simulink model "Impcont_foot"  (R2016a)
settings: Solver=ode23tb  StartTime=0.0  StopTime=ti(end)  MaxStep=1e-3
InitFcn:
  | fp_sp_k = 12e3;
  | fp_sp_d = 1;
  | weights = 70/6;
  | joint_k = 0.1*180/pi;
  | joint_d = 1*180/pi;
  | fp_uj_dp_k = 500*180/pi;
  | fp_uj_dp_d = 1*180/pi;
  | fp_uj_ie_k = 500*180/pi;
  | fp_uj_ie_d = 1*180/pi;
  | 
  | x_k = 0*180/pi; x_d = 0.5*180/pi;
  | y_k = 0*180/pi; y_d = 0.5*180/pi;
  | z_k = 0*180/pi; z_d = 0.5*180/pi;
  | 
  | %{
  | stiff_dp=0.1*180/pi; stiff_ie=1*180/pi;
  | damp_dp=1*180/pi; damp_ie=1*180/pi;
  | % offset of prosthesis from centre of FP (XZY)
  |  sta=[-0.5345-6.54e-2 0.03779 0];
  | %}
  | 
  | % initpos = inv(jacob_gaitEmul(zeros(6,1)))*[ankle.trans(1,:).'; zeros(3,1)];
  | 
  | % sta = -[initpos(1) initpos(2) initpos(3)];
StopFcn:
  | %{
  | ankle = struct('ang_dp', angle_dp_out.signals.values,'ang_ie', angle_ie_out.signals.values,...
  |            'vel_dp',vel_dp.signals.values,'vel_ie',vel_ie.signals.values,...
  |            'acc_dp',acc_dp.signals.values,'acc_ie',acc_ie.signals.values,...
  |            'trans',ankle_trans_out.signals.values);
  | shin = struct('trans', trans_shin.signals.values, 'quat', quat_shin.signals.values);
  | foot = struct('trans', trans_foot.signals.values, 'quat', quat_foot.signals.values,...
  |     'acc',acc_foot.signals.values);
  | fplate = struct('trans', trans_fp.signals.values, 'quat', quat_fp.signals.values,...
  |     'torques', fp_torque_out.signals.values, 'forces', fp_force_out.signals.values);
  | 
  | [~, ~, ankle_ej.trans, ~] = est_joint(shin, foot);
  | 
  | fpForce = quatrotate(quatinv(fplate.quat), fplate.forces);
  | fpTorque = quatrotate(quatinv(fplate.quat), fplate.torques);
  | 
  | torque = cross(fplate.trans - ankle_ej.trans, fpForce) + fpTorque;
  | 
  | regMdl_dp = regress(torque(:,3),[ankle.ang_dp ankle.vel_dp foot.acc(:,3)]);
  | regMdl_ie = regress(torque(:,1),[ankle.ang_ie ankle.vel_ie foot.acc(:,1)]);
  | analysis_si = struct('kdp',regMdl_dp(1),'bdp',regMdl_dp(2),...
  |     'kie',regMdl_ie(1),'bie',regMdl_ie(2),'Jdp',regMdl_dp(3),...
  |     'Jie',regMdl_ie(3));
  | 
  | % %{
  | regMdl_dp = regress(torque(:,3),[ankle.ang_dp ankle.vel_dp ankle.acc_dp]);
  | regMdl_ie = regress(torque(:,1),[ankle.ang_ie ankle.vel_ie ankle.acc_ie]);
  | analysis_si2 = struct('kdp',regMdl_dp(1),'bdp',regMdl_dp(2),...
  |     'kie',regMdl_ie(1),'bie',regMdl_ie(2),'Jdp',regMdl_dp(3),...
  |     'Jie',regMdl_ie(3));
  | % %}
  | 
  | % %{
  | regMdl_dp = regress(tt_dp.signals.values(:,3),[ankle.ang_dp ankle.vel_dp ankle.acc_dp]);
  | regMdl_ie = regress(tt_ie.signals.values(:,3),[ankle.ang_ie ankle.vel_ie ankle.acc_ie]);
  | analysis_si3 = struct('kdp',regMdl_dp(1),'bdp',regMdl_dp(2),...
  |     'kie',regMdl_ie(1),'bie',regMdl_ie(2),'Jdp',regMdl_dp(3),...
  |     'Jie',regMdl_ie(3));
  | % %}
  | 
  | % %{
  | regMdl_dp = regress(tt_dp.signals.values(:,3),[ankle.ang_dp ankle.vel_dp foot.acc(:,3)]);
  | regMdl_ie = regress(tt_ie.signals.values(:,3),[ankle.ang_ie ankle.vel_ie foot.acc(:,1)]);
  | analysis_si4 = struct('kdp',regMdl_dp(1),'bdp',regMdl_dp(2),...
  |     'kie',regMdl_ie(1),'bie',regMdl_ie(2),'Jdp',regMdl_dp(3),...
  |     'Jie',regMdl_ie(3));
  | % %}
  | 
  | regMdl_dp = regress(torque(:,3),[ankle.ang_dp ankle.vel_dp]);
  | regMdl_ie = regress(torque(:,1),[ankle.ang_ie ankle.vel_ie]);
  | analysis_si5 = struct('kdp',regMdl_dp(1),'bdp',regMdl_dp(2),...
  |     'kie',regMdl_ie(1),'bie',regMdl_ie(2));
  | 
  | %}
values from neighbouring files (symbols this model uses):
  N = length(shin_angles_in.signals.values)    [GaitEmu_code.m]    (also in dy1.m; dy2.m; est_joint.m = size( [body1.trans body2.trans], 1 ); impcont.m)
  s = [-atan((t2.*3.379e-4+t3+t4.*t5.*4.401e-2)./(t4.*cos(q2)));-asin(t2.*1.4870979e-5+t3.*4.401e-2-t4.*t5)]    [FK_af.m]    (also in FK_footimp.m = [atan((ree2_1.*t2.*4.401e-2+ree2_2.*t4+ree2_3.*t3+t5.*t7.*4.; FK_gaitEmul.m = [q1+t2.*t4.*4.234e-1+t3.*t5.*1.5e-3-t2.*t6.*t7.*1.5e-3-5.347; ik.m = [x; y; z]; ik_af.m = FK_af(q))
  Y = -( reshape( body1.trans', [], 1 ) - reshape( body2.trans', [], 1 ) )    [creat_joint.m]    (also in est_joint.m = -( reshape( body1.trans', [3*N 1] ) - reshape( body2.trans',)
undefined symbols (not defined in the file or in its folder): X, Z
libraries: sm_lib x274, nesl_utility x100, simulink x3, dspstat3 x2, aerolibtransform2 x1
(part 1 of 7)
settings Model: Creator=lcasteli  LastModifiedBy=lcasteli
settings SolverCC: ZeroCrossControl=DisableAll  AlgebraicLoopSolver=LineSearch
settings DataIOCC: OutputTimes=[0:0.01:t(end)]
settings ModelReferenceCC: ModelReferenceMinAlgLoopOccurrences=on

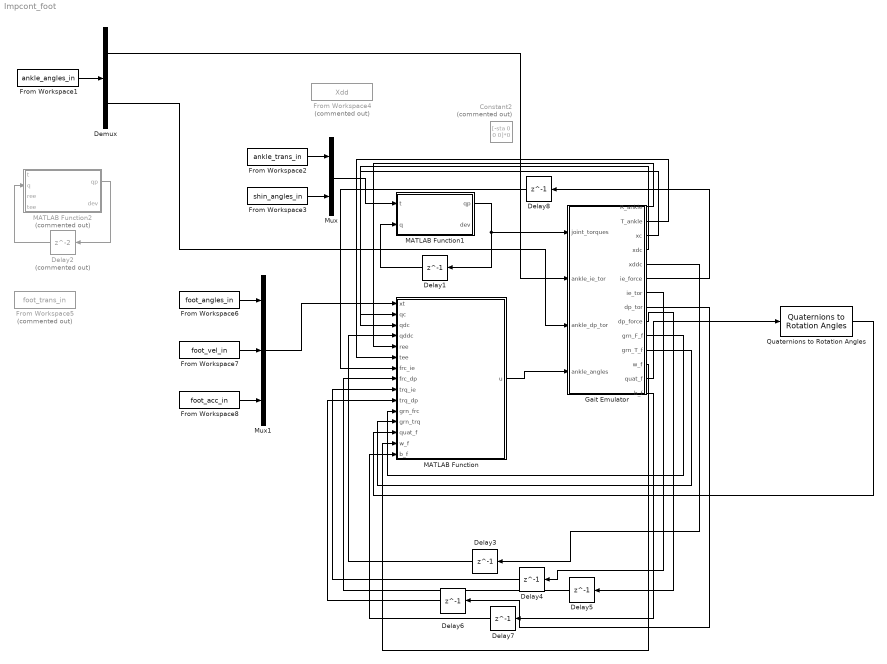
== system Impcont_foot ==
  Constant2 : Constant  Commented=on  Value=[-sta 0 0 0]*0
  Delay{1,3..8} (7 alike) : Delay  DelayLength=1  SampleTime=0.01
  Delay2 : Delay  Commented=on  SampleTime=0.01
  Demux : Demux  Outputs=2
  From Workspace1 : FromWorkspace  VariableName=ankle_angles_in  SampleTime=0
  From Workspace2 : FromWorkspace  VariableName=ankle_trans_in  SampleTime=0
  From Workspace3 : FromWorkspace  VariableName=shin_angles_in  SampleTime=0
  From Workspace4 : FromWorkspace  Commented=on  VariableName=Xdd  SampleTime=0
  From Workspace5 : FromWorkspace  Commented=on  VariableName=foot_trans_in  SampleTime=0
  From Workspace6 : FromWorkspace  VariableName=foot_angles_in  SampleTime=0
  From Workspace7 : FromWorkspace  VariableName=foot_vel_in  SampleTime=0
  From Workspace8 : FromWorkspace  VariableName=foot_acc_in  SampleTime=0
  Gait Emulator : Subsystem
  MATLAB Function : MATLAB Function  TreatAsAtomicUnit=on
  MATLAB Function1 : MATLAB Function  TreatAsAtomicUnit=on
  MATLAB Function2 : MATLAB Function  Commented=on  TreatAsAtomicUnit=on
  Mux : Mux  Inputs=2
  Mux1 : Mux  Inputs=3
  Quaternions to Rotation Angles : aerolibtransform2/Quaternions to Rotation Angles  rotationOrder=XYZ
  wires:
  Delay1/1 -> MATLAB Function1/2(q)
  MATLAB Function1/1(qp) -> Delay1/1, Gait Emulator/1(joint_torques)
  From Workspace1/1 -> Demux/1
  From Workspace2/1 -> Mux/1
  From Workspace3/1 -> Mux/2
  Mux/1 -> MATLAB Function1/1(t)
  Gait Emulator/2(T_ankle) -> MATLAB Function/6(tee)
  Gait Emulator/1(R_ankle) -> MATLAB Function/5(ree)
  Gait Emulator/3(xc) -> MATLAB Function/2(qc)
  Gait Emulator/4(xdc) -> MATLAB Function/3(qdc)
  Gait Emulator/5(xddc) -> Delay3/1
  Gait Emulator/6(ie_force) -> Delay8/1
  Gait Emulator/7(ie_tor) -> Delay4/1
  Gait Emulator/9(dp_force) -> Delay5/1
  Gait Emulator/8(dp_tor) -> Delay6/1
  MATLAB Function2/1(qp) -> Delay2/1
  Delay2/1 -> MATLAB Function2/2(q)
  From Workspace8/1 -> Mux1/3
  From Workspace7/1 -> Mux1/2
  From Workspace6/1 -> Mux1/1
  Mux1/1 -> MATLAB Function/1(xt)
  MATLAB Function/1(u) -> Gait Emulator/4(ankle_angles)
  Gait Emulator/10(grn_F_f) -> MATLAB Function/11(grn_frc)
  Gait Emulator/11(grn_T_f) -> MATLAB Function/12(grn_trq)
  Gait Emulator/14(b_f) -> Delay7/1
  Gait Emulator/13(quat_f) -> Quaternions to Rotation Angles/1
  Quaternions to Rotation Angles/1 -> MATLAB Function/13(quat_f)
  Delay3/1 -> MATLAB Function/4(qddc)
  Delay4/1 -> MATLAB Function/9(trq_ie)
  Delay5/1 -> MATLAB Function/8(frc_dp)
  Delay6/1 -> MATLAB Function/10(trq_dp)
  Delay7/1 -> MATLAB Function/15(b_f)
  Gait Emulator/12(w_f) -> MATLAB Function/14(w_f)
  Delay8/1 -> MATLAB Function/7(frc_ie)
  Demux/1 -> Gait Emulator/2(ankle_ie_tor)
  Demux/2 -> Gait Emulator/3(ankle_dp_tor)

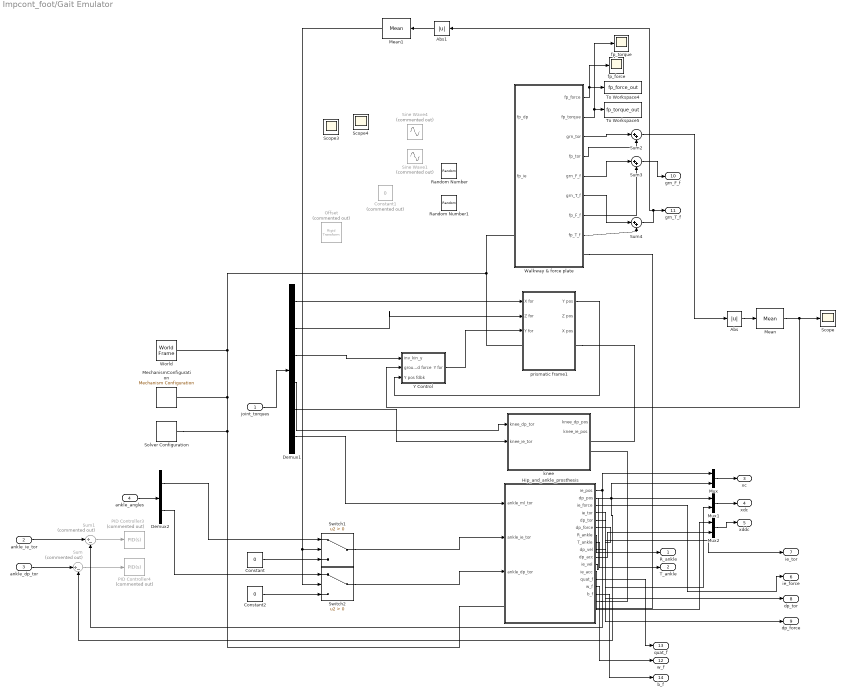
== system Impcont_foot/Gait Emulator ==
  joint_torques : Inport
  ankle_ie_tor : Inport  Port=2
  ankle_dp_tor : Inport  Port=3
  ankle_angles : Inport  Port=4
  Abs : Abs
  Abs1 : Abs
  Constant : Constant  Value=0
  Constant1 : Constant  Commented=on  Value=0
  Constant2 : Constant  Value=0
  Demux1 : Demux  Outputs=6
  Demux2 : Demux  Outputs=2
  Hip_and_ankle_prosthesis : Subsystem
  Mean : dspstat3/Mean  run=off  reset_popup=None  InputProcessing=Columns as channels (frame based)  directionMode=Each column  dimension=1  roiEnable=off  roiType=Rectangles  roiPortion=Entire ROI  roiOutput=Individual statistics for each ROI  roiFlag=off  outputDataTypeStr=Inherit: Same as accumulator  outputLastDataTypeStr=Inherit: Same as accumulator  outputMin=[]  outputMax=[]  roundingMode=Floor  overflowMode=off
  Mean1 : dspstat3/Mean  run=off  reset_popup=None  InputProcessing=Columns as channels (frame based)  directionMode=Each column  dimension=1  roiEnable=off  roiType=Rectangles  roiPortion=Entire ROI  roiOutput=Individual statistics for each ROI  roiFlag=off  outputDataTypeStr=Inherit: Same as accumulator  outputLastDataTypeStr=Inherit: Same as accumulator  outputMin=[]  outputMax=[]  roundingMode=Floor  overflowMode=off
  MechanismConfiguration : sm_lib/Utilities/Mechanism Configuration  UniformGravity=Constant  GravityVector=[0 -9.81 0]  GravityUnits=m/s^2  LinearizationDelta=0.001
  Mux : Mux  Inputs=2
  Mux1 : Mux  Inputs=2
  Mux2 : Mux  Inputs=2
  Offset : sm_lib/Frames and Transforms/Rigid Transform  Commented=on  TranslationMethod=Cartesian  TranslationLengthUnit=m  TranslationStandardAxis=+Z  TranslationStandardOffset=0  TranslationCartesianOffset=[0.5345 0 -0.03779]  TranslationROffset=0  TranslationROffsetUnits=m  TranslationZOffset=0  TranslationZOffsetUnits=m  TranslationThetaOffset=0  TranslationThetaOffsetUnits=deg  RotationMethod=None  RotationAngleUnits=deg  RotationStandardAxis=+Z  RotationAngle=0.0  RotationArbitraryAxis=[0 0 1]  FollAlignAxisA=+X  BaseAlignAxisA=+Y  FollAlignAxisB=+Y  BaseAlignAxisB=+Z  RotationSequenceAxes=FollowerAxes  RotationSequence=XYX  RotationSequenceAngles=[0 0 0]  RotationSequenceAnglesUnits=deg  RotationMatrix=[1 0 0; 0 1 0; 0 0 1]
  PID Controller3 : simulink/Continuous/PID Controller  Commented=on  Controller=PID  TimeDomain=Continuous-time  SampleTime=-1  IntegratorMethod=Forward Euler  FilterMethod=Forward Euler  Form=Parallel  UseFilter=on  ControllerParametersSource=internal  P=975.875057621142  I=4739.46701283172  D=-0.483288607910801  N=2019.23869432746  InitialConditionSource=internal  InitialConditionForIntegrator=0  InitialConditionForFilter=0  ExternalReset=none  LimitOutput=off  UpperSaturationLimit=300  LowerSaturationLimit=-300  LinearizeAsGain=on  AntiWindupMode=clamping  Kb=1  TrackingMode=off  Kt=1  PParamMin=[]  PParamMax=[]  IParamMin=[]  IParamMax=[]  DParamMin=[]  DParamMax=[]  NParamMin=[]  NParamMax=[]  KbParamMin=[]  KbParamMax=[]  KtParamMin=[]  KtParamMax=[]  POutMin=[]  POutMax=[]  IOutMin=[]  IOutMax=[]  DOutMin=[]  DOutMax=[]  NOutMin=[]  NOutMax=[]  KbOutMin=[]  KbOutMax=[]  KtOutMin=[]  KtOutMax=[]  IntegratorOutMin=[]  IntegratorOutMax=[]  FilterOutMin=[]  FilterOutMax=[]  SumOutMin=[]  SumOutMax=[]  SumI1OutMin=[]  SumI1OutMax=[]  SumI2OutMin=[]  SumI2OutMax=[]  SumI3OutMin=[]  SumI3OutMax=[]  SumDOutMin=[]  SumDOutMax=[]  SaturationOutMin=[]  SaturationOutMax=[]  IntegratorContinuousStateAttributes=''  IntegratorStateMustResolveToSignalObject=off  IntegratorRTWStateStorageClass=Auto  FilterContinuousStateAttributes=''  FilterStateMustResolveToSignalObject=off  FilterRTWStateStorageClass=Auto  DifferentiatorICPrevScaledInput=0  DifferentiatorOutMin=[]  DifferentiatorOutMax=[]
  PID Controller4 : simulink/Continuous/PID Controller  Commented=on  Controller=PID  TimeDomain=Continuous-time  SampleTime=-1  IntegratorMethod=Forward Euler  FilterMethod=Forward Euler  Form=Parallel  UseFilter=on  ControllerParametersSource=internal  P=1292.14032707455  I=5309.73525196698  D=-11.9075203483279  N=25.559430935789  InitialConditionSource=internal  InitialConditionForIntegrator=0  InitialConditionForFilter=0  ExternalReset=none  LimitOutput=off  UpperSaturationLimit=300  LowerSaturationLimit=-300  LinearizeAsGain=on  AntiWindupMode=clamping  Kb=1  TrackingMode=off  Kt=1  PParamMin=[]  PParamMax=[]  IParamMin=[]  IParamMax=[]  DParamMin=[]  DParamMax=[]  NParamMin=[]  NParamMax=[]  KbParamMin=[]  KbParamMax=[]  KtParamMin=[]  KtParamMax=[]  POutMin=[]  POutMax=[]  IOutMin=[]  IOutMax=[]  DOutMin=[]  DOutMax=[]  NOutMin=[]  NOutMax=[]  KbOutMin=[]  KbOutMax=[]  KtOutMin=[]  KtOutMax=[]  IntegratorOutMin=[]  IntegratorOutMax=[]  FilterOutMin=[]  FilterOutMax=[]  SumOutMin=[]  SumOutMax=[]  SumI1OutMin=[]  SumI1OutMax=[]  SumI2OutMin=[]  SumI2OutMax=[]  SumI3OutMin=[]  SumI3OutMax=[]  SumDOutMin=[]  SumDOutMax=[]  SaturationOutMin=[]  SaturationOutMax=[]  IntegratorContinuousStateAttributes=''  IntegratorStateMustResolveToSignalObject=off  IntegratorRTWStateStorageClass=Auto  FilterContinuousStateAttributes=''  FilterStateMustResolveToSignalObject=off  FilterRTWStateStorageClass=Auto  DifferentiatorICPrevScaledInput=0  DifferentiatorOutMin=[]  DifferentiatorOutMax=[]
  Random Number : RandomNumber  Variance=4e5  SampleTime=0.1
  Random Number1 : RandomNumber  Variance=1e4  SampleTime=0.1
  Scope : Scope
  Scope3 : Scope
  Scope4 : Scope
  Sine Wave1 : Sin  Commented=on  Amplitude=100  Frequency=10  Phase=pi/6  SampleTime=0.001
  Sine Wave4 : Sin  Commented=on  Amplitude=100*2  Frequency=10  SampleTime=0.001
  Solver Configuration : nesl_utility/Solver Configuration  PhysicalDomain=network_engine_domain  SubClassName=solver  LeftPortType=input  RightPortType=generic  Accelerate=off  Tones=[]  Harmonics=[]  SimulateNoise=off  Profile=off  UseLocalSampling=off  EnableSwitchedLinearOptims=on  FrequencyDomain=off  UseCCode=off  RelTol=0.001  AbsTol=1e-06  MinStep=1e-09  ToWorkspace=off  RevertToSquareIcSolve=off  NumHomotopyIterations=100  PhasorMode=off  PhasorModeNumHarmonics=1  OverrideAbsTol=off  DoDC=off  ResidualTolerance=1e-09  UseLocalSolver=off  LocalSolverChoice=NE_BACKWARD_EULER_ADVANCER  LocalSolverSampleTime=0.001  DoFixedCost=off  MaxNonlinIter=3  MaxModeIter=2  LinearAlgebra=Sparse  DelaysMemoryBudget=1024  AutomaticFiltering=on  FilteringTimeConstant=0.001
  Sum : Sum  Commented=on  Inputs=|+-
  Sum1 : Sum  Commented=on  Inputs=|+-
  Sum2 : Sum  Inputs=|++
  Sum3 : Sum  Inputs=|++
  Sum4 : Sum  Inputs=|++
  Switch1 : Switch  Criteria=u2 > Threshold
  Switch2 : Switch  Criteria=u2 > Threshold
  To Workspace4 : ToWorkspace  VariableName=fp_force_out  SaveFormat=Structure With Time  SampleTime=-1
  To Workspace5 : ToWorkspace  VariableName=fp_torque_out  SaveFormat=Structure With Time  SampleTime=-1
  Walkway & force plate : Subsystem
  World : sm_lib/Frames and Transforms/World Frame
  Y Control : Subsystem
  fp_force : Scope
  fp_torque : Scope
  "knee " : Subsystem
  prismatic frame1 : Subsystem
  R_ankle : Outport
  T_ankle : Outport  Port=2
  xc : Outport  Port=3
  xdc : Outport  Port=4
  xddc : Outport  Port=5
  ie_force : Outport  Port=6
  ie_tor : Outport  Port=7
  dp_tor : Outport  Port=8
  dp_force : Outport  Port=9
  grn_F_f : Outport  Port=10
  grn_T_f : Outport  Port=11
  w_f : Outport  Port=12
  quat_f : Outport  Port=13
  b_f : Outport  Port=14
  wires:
  joint_torques/1 -> Demux1/1
  Walkway & force plate/2(fp_torque) -> fp_torque/1, To Workspace5/1
  Walkway & force plate/1(fp_force) -> To Workspace4/1, fp_force/1
  Demux1/4 -> "knee "/1(knee_dp_tor)
  Demux1/5 -> "knee "/2(knee_ie_tor)
  Demux1/6 -> Hip_and_ankle_prosthesis/1(ankle_ml_tor)
  Walkway & force plate/3(grn_tor) -> Sum2/1
  Walkway & force plate/4(fp_tor) -> Sum2/2
  Sum2/1 -> Abs/1
  Abs/1 -> Mean/1
  Mean/1 -> Y Control/2(ground force), Scope/1
  Hip_and_ankle_prosthesis/2(dp_pos) -> Sum/2, Mux/2
  Sum1/1 -> PID Controller3/1
  Sum/1 -> PID Controller4/1
  Demux1/1 -> prismatic frame1/1(X for)
  prismatic frame1/1(Y pos) -> Y Control/3(Y pos fdbk)
  Demux1/2 -> prismatic frame1/2(Z for)
  Demux1/3 -> Y Control/1(inv_kin_y)
  Y Control/1(Y for) -> prismatic frame1/3(Y for)
  ankle_ie_tor/1 -> Sum1/1
  ankle_dp_tor/1 -> Sum/1
  Hip_and_ankle_prosthesis/8(T_ankle) -> T_ankle/1
  Hip_and_ankle_prosthesis/7(R_ankle) -> R_ankle/1
  ankle_angles/1 -> Demux2/1
  Hip_and_ankle_prosthesis/1(ie_pos) -> Sum1/2, Mux/1
  Hip_and_ankle_prosthesis/11(ie_vel) -> Mux1/1
  Hip_and_ankle_prosthesis/9(dp_vel) -> Mux1/2
  Hip_and_ankle_prosthesis/12(ie_acc) -> Mux2/1
  Hip_and_ankle_prosthesis/10(dp_acc) -> Mux2/2
  Mux2/1 -> xddc/1
  Mux1/1 -> xdc/1
  Mux/1 -> xc/1
  Hip_and_ankle_prosthesis/3(ie_force) -> ie_force/1
  Hip_and_ankle_prosthesis/4(ie_tor) -> ie_tor/1
  Hip_and_ankle_prosthesis/6(dp_force) -> dp_force/1
  Hip_and_ankle_prosthesis/5(dp_tor) -> dp_tor/1
  Sum3/1 -> grn_F_f/1
  Hip_and_ankle_prosthesis/13(quat_f) -> quat_f/1
  Hip_and_ankle_prosthesis/14(w_f) -> w_f/1
  Hip_and_ankle_prosthesis/15(b_f) -> b_f/1
  Walkway & force plate/7(fp_F_f) -> Sum3/2
  Walkway & force plate/5(grn_F_f) -> Sum3/1
  Walkway & force plate/8(fp_T_f) -> Sum4/2
  Walkway & force plate/6(grn_T_f) -> Sum4/1
  Sum4/1 -> grn_T_f/1, Abs1/1
  Demux2/1 -> Switch1/1
  Demux2/2 -> Switch2/1
  Switch1/1 -> Hip_and_ankle_prosthesis/2(ankle_ie_tor)
  Switch2/1 -> Hip_and_ankle_prosthesis/3(ankle_dp_tor)
  Abs1/1 -> Mean1/1
  Mean1/1 -> Switch2/2, Switch1/2
  Constant2/1 -> Switch2/3
  Constant/1 -> Switch1/3
  connections:
  Hip_and_ankle_prosthesis/RConn1 -- "knee "/RConn2
  Walkway & force plate/RConn1 -- Hip_and_ankle_prosthesis/RConn2
  prismatic frame1/LConn1 -- Walkway & force plate/LConn1 -- Hip_and_ankle_prosthesis/LConn1 -- Solver Configuration/RConn1 -- MechanismConfiguration/RConn1 -- World/RConn1
  prismatic frame1/RConn1 -- "knee "/RConn1

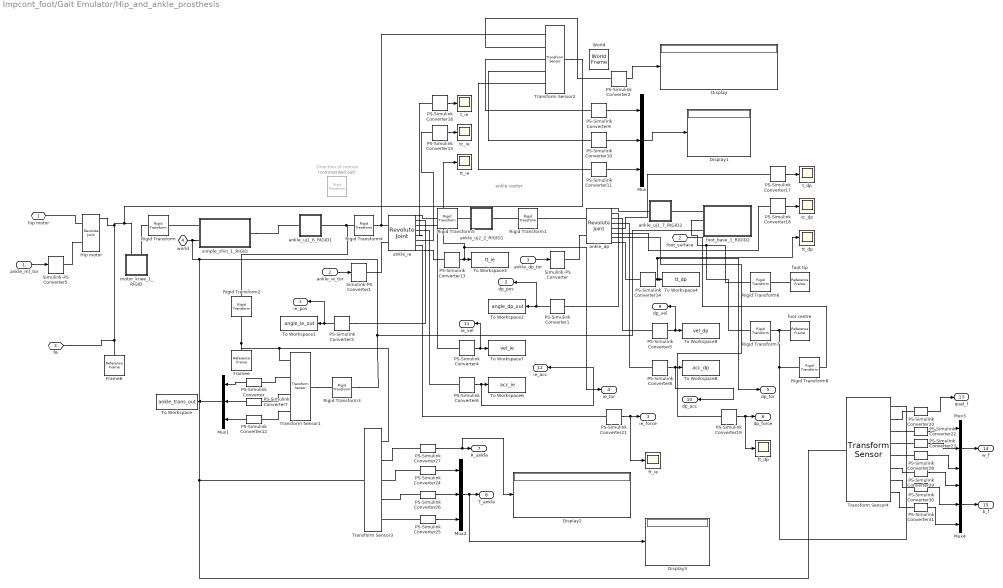
== system Impcont_foot/Gait Emulator/Hip_and_ankle_prosthesis ==
  note: ankle center
  ankle_ml_tor : Inport
  ankle_ie_tor : Inport  Port=2
  ankle_dp_tor : Inport  Port=3
  Display{,1..3} (4 alike) : Display
  Driection of motion : sm_lib/Frames and Transforms/Rigid Transform  Commented=on  TranslationMethod=None  TranslationLengthUnit=m  TranslationStandardAxis=+Z  TranslationStandardOffset=0  TranslationCartesianOffset=[0 0 0]  TranslationROffset=0  TranslationROffsetUnits=m  TranslationZOffset=0  TranslationZOffsetUnits=m  TranslationThetaOffset=0  TranslationThetaOffsetUnits=deg  RotationMethod=StandardAxis  RotationAngleUnits=deg  RotationStandardAxis=+Z  RotationAngle=0  RotationArbitraryAxis=[0 0 1]  FollAlignAxisA=+X  BaseAlignAxisA=+Y  FollAlignAxisB=+Y  BaseAlignAxisB=+Z  RotationSequenceAxes=FollowerAxes  RotationSequence=XYX  RotationSequenceAngles=[0 0 0]  RotationSequenceAnglesUnits=deg  RotationMatrix=[1 0 0; 0 1 0; 0 0 1]
  Frame6 : sm_lib/Frames and Transforms/Reference Frame
  Framee : sm_lib/Frames and Transforms/Reference Frame
  Hip motor : sm_lib/Joints/Revolute Joint  SenseConstraintForce=off  SenseConstraintForceX=off  SenseConstraintForceY=off  SenseConstraintForceZ=off  SenseConstraintTorque=off  SenseConstraintTorqueX=off  SenseConstraintTorqueY=off  SenseConstraintTorqueZ=off  SenseTotalForce=on  SenseTotalForceX=off  SenseTotalForceY=off  SenseTotalForceZ=off  SenseTotalTorque=on  SenseTotalTorqueX=off  SenseTotalTorqueY=off  SenseTotalTorqueZ=off  CompositeWrenchDir=FollowerOnBase  CompositeWrenchFrame=BaseFrame  EquilibriumPosition=0  EquilibriumPositionUnits=rad  SpringStiffness=joint_k  SpringStiffnessUnits=m*N/rad  DampingCoefficient=joint_d  DampingCoefficientUnits=m*s*N/rad  TorqueActuationMode=ComputedTorque  MotionActuationMode=InputMotion  SensePosition=on  SenseVelocity=off  SenseAcceleration=off  SenseTorqueForce=off  PositionTargetSpecify=off  PositionTargetPriority=Low  PositionTargetValue=0  PositionTargetValueUnits=deg  VelocityTargetSpecify=off  VelocityTargetPriority=High  VelocityTargetValue=0  VelocityTargetValueUnits=deg/s
  Mux{,1..4} (5 alike) : Mux  Inputs=3
  PS-Simulink Converter{,1..31} (32 alike) : nesl_utility/PS-Simulink Converter  PhysicalDomain=network_engine_domain  SubClassName=ps_output  LeftPortType=input  RightPortType=output  PseudoPeriodic=off  Frequencies=[]  Unit=1  AffineConversion=off
  Rigid Transform : sm_lib/Frames and Transforms/Rigid Transform  TranslationMethod=StandardAxis  TranslationLengthUnit=m  TranslationStandardAxis=+Z  TranslationStandardOffset=0.15  TranslationCartesianOffset=[0 0 0]  TranslationROffset=0  TranslationROffsetUnits=m  TranslationZOffset=0  TranslationZOffsetUnits=m  TranslationThetaOffset=0  TranslationThetaOffsetUnits=deg  RotationMethod=StandardAxis  RotationAngleUnits=deg  RotationStandardAxis=+X  RotationAngle=180  RotationArbitraryAxis=[1 0 1]  FollAlignAxisA=+X  BaseAlignAxisA=+Y  FollAlignAxisB=+Y  BaseAlignAxisB=+Z  RotationSequenceAxes=FollowerAxes  RotationSequence=XYX  RotationSequenceAngles=[0 0 0]  RotationSequenceAnglesUnits=deg  RotationMatrix=[1 0 0; 0 1 0; 0 0 1]
  Rigid Transform1 : sm_lib/Frames and Transforms/Rigid Transform  TranslationMethod=None  TranslationLengthUnit=m  TranslationStandardAxis=+Z  TranslationStandardOffset=0.15  TranslationCartesianOffset=[0 0 0]  TranslationROffset=0  TranslationROffsetUnits=m  TranslationZOffset=0  TranslationZOffsetUnits=m  TranslationThetaOffset=0  TranslationThetaOffsetUnits=deg  RotationMethod=StandardAxis  RotationAngleUnits=deg  RotationStandardAxis=+Z  RotationAngle=-90  RotationArbitraryAxis=[1 0 1]  FollAlignAxisA=+X  BaseAlignAxisA=+Y  FollAlignAxisB=+Y  BaseAlignAxisB=+Z  RotationSequenceAxes=FollowerAxes  RotationSequence=XYX  RotationSequenceAngles=[0 0 0]  RotationSequenceAnglesUnits=deg  RotationMatrix=[1 0 0; 0 1 0; 0 0 1]
  Rigid Transform2 : sm_lib/Frames and Transforms/Rigid Transform  TranslationMethod=StandardAxis  TranslationLengthUnit=m  TranslationStandardAxis=+Z  TranslationStandardOffset=-8.5e-3  TranslationCartesianOffset=[0 0 0]  TranslationROffset=0  TranslationROffsetUnits=m  TranslationZOffset=0  TranslationZOffsetUnits=m  TranslationThetaOffset=0  TranslationThetaOffsetUnits=deg  RotationMethod=AlignedAxes  RotationAngleUnits=deg  RotationStandardAxis=+Z  RotationAngle=-90  RotationArbitraryAxis=[1 0 1]  FollAlignAxisA=+X  BaseAlignAxisA=-Z  FollAlignAxisB=+Y  BaseAlignAxisB=-Y  RotationSequenceAxes=FollowerAxes  RotationSequence=XYX  RotationSequenceAngles=[0 0 0]  RotationSequenceAnglesUnits=deg  RotationMatrix=[1 0 0; 0 1 0; 0 0 1]
  Rigid Transform3 : sm_lib/Frames and Transforms/Rigid Transform  TranslationMethod=StandardAxis  TranslationLengthUnit=m  TranslationStandardAxis=+Y  TranslationStandardOffset=0.1517  TranslationCartesianOffset=[0 0 0]  TranslationROffset=0  TranslationROffsetUnits=m  TranslationZOffset=0  TranslationZOffsetUnits=m  TranslationThetaOffset=0  TranslationThetaOffsetUnits=deg  RotationMethod=None  RotationAngleUnits=deg  RotationStandardAxis=+Z  RotationAngle=0.0  RotationArbitraryAxis=[0 0 1]  FollAlignAxisA=+X  BaseAlignAxisA=+Y  FollAlignAxisB=+Y  BaseAlignAxisB=+Z  RotationSequenceAxes=FollowerAxes  RotationSequence=XYX  RotationSequenceAngles=[0 0 0]  RotationSequenceAnglesUnits=deg  RotationMatrix=[1 0 0; 0 1 0; 0 0 1]
  Rigid Transform4 : sm_lib/Frames and Transforms/Rigid Transform  TranslationMethod=StandardAxis  TranslationLengthUnit=m  TranslationStandardAxis=+Z  TranslationStandardOffset=-8.5e-3  TranslationCartesianOffset=[0 0 0]  TranslationROffset=0  TranslationROffsetUnits=m  TranslationZOffset=0  TranslationZOffsetUnits=m  TranslationThetaOffset=0  TranslationThetaOffsetUnits=deg  RotationMethod=None  RotationAngleUnits=deg  RotationStandardAxis=+Z  RotationAngle=0.0  RotationArbitraryAxis=[0 0 1]  FollAlignAxisA=+X  BaseAlignAxisA=+Y  FollAlignAxisB=+Y  BaseAlignAxisB=+Z  RotationSequenceAxes=FollowerAxes  RotationSequence=XYX  RotationSequenceAngles=[0 0 0]  RotationSequenceAnglesUnits=deg  RotationMatrix=[1 0 0; 0 1 0; 0 0 1]
  Rigid Transform5 : sm_lib/Frames and Transforms/Rigid Transform  TranslationMethod=StandardAxis  TranslationLengthUnit=m  TranslationStandardAxis=+Z  TranslationStandardOffset=8.5e-3  TranslationCartesianOffset=[0 0 0]  TranslationROffset=0  TranslationROffsetUnits=m  TranslationZOffset=0  TranslationZOffsetUnits=m  TranslationThetaOffset=0  TranslationThetaOffsetUnits=deg  RotationMethod=None  RotationAngleUnits=deg  RotationStandardAxis=+Z  RotationAngle=0.0  RotationArbitraryAxis=[0 0 1]  FollAlignAxisA=+X  BaseAlignAxisA=+Y  FollAlignAxisB=+Y  BaseAlignAxisB=+Z  RotationSequenceAxes=FollowerAxes  RotationSequence=XYX  RotationSequenceAngles=[0 0 0]  RotationSequenceAnglesUnits=deg  RotationMatrix=[1 0 0; 0 1 0; 0 0 1]
  Rigid Transform6 : sm_lib/Frames and Transforms/Rigid Transform  TranslationMethod=StandardAxis  TranslationLengthUnit=m  TranslationStandardAxis=+X  TranslationStandardOffset=-0.181  TranslationCartesianOffset=[0 0 0]  TranslationROffset=0  TranslationROffsetUnits=m  TranslationZOffset=0  TranslationZOffsetUnits=m  TranslationThetaOffset=0  TranslationThetaOffsetUnits=deg  RotationMethod=None  RotationAngleUnits=deg  RotationStandardAxis=+Z  RotationAngle=0.0  RotationArbitraryAxis=[0 0 1]  FollAlignAxisA=+X  BaseAlignAxisA=+Y  FollAlignAxisB=+Y  BaseAlignAxisB=+Z  RotationSequenceAxes=FollowerAxes  RotationSequence=XYX  RotationSequenceAngles=[0 0 0]  RotationSequenceAnglesUnits=deg  RotationMatrix=[1 0 0; 0 1 0; 0 0 1]
  Rigid Transform7 : sm_lib/Frames and Transforms/Rigid Transform  TranslationMethod=StandardAxis  TranslationLengthUnit=m  TranslationStandardAxis=+X  TranslationStandardOffset=-0.181/2  TranslationCartesianOffset=[0 0 0]  TranslationROffset=0  TranslationROffsetUnits=m  TranslationZOffset=0  TranslationZOffsetUnits=m  TranslationThetaOffset=0  TranslationThetaOffsetUnits=deg  RotationMethod=StandardAxis  RotationAngleUnits=deg  RotationStandardAxis=+X  RotationAngle=90  RotationArbitraryAxis=[0 0 1]  FollAlignAxisA=+X  BaseAlignAxisA=+Y  FollAlignAxisB=+Y  BaseAlignAxisB=+Z  RotationSequenceAxes=FollowerAxes  RotationSequence=XYX  RotationSequenceAngles=[0 0 0]  RotationSequenceAnglesUnits=deg  RotationMatrix=[1 0 0; 0 1 0; 0 0 1]
  Rigid Transform8 : sm_lib/Frames and Transforms/Rigid Transform  TranslationMethod=None  TranslationLengthUnit=m  TranslationStandardAxis=+X  TranslationStandardOffset=-0.181/2  TranslationCartesianOffset=[0 0 0]  TranslationROffset=0  TranslationROffsetUnits=m  TranslationZOffset=0  TranslationZOffsetUnits=m  TranslationThetaOffset=0  TranslationThetaOffsetUnits=deg  RotationMethod=StandardAxis  RotationAngleUnits=deg  RotationStandardAxis=+X  RotationAngle=-90  RotationArbitraryAxis=[0 0 1]  FollAlignAxisA=+X  BaseAlignAxisA=+Y  FollAlignAxisB=+Y  BaseAlignAxisB=+Z  RotationSequenceAxes=FollowerAxes  RotationSequence=XYX  RotationSequenceAngles=[0 0 0]  RotationSequenceAnglesUnits=deg  RotationMatrix=[1 0 0; 0 1 0; 0 0 1]
  Simulink-PS Converter : nesl_utility/Simulink-PS Converter  PhysicalDomain=network_engine_domain  SubClassName=ps_input  LeftPortType=input  RightPortType=output  PseudoPeriodic=off  Frequencies=[]  NoiseDistribution=none  NoiseParameters=[]  Unit=1  AffineConversion=off  InputFiltering=on  SimscapeFilterOrder=2  InputFilterTimeConstant=0.001  UdotUserProvided=1
  Simulink-PS Converter1 : nesl_utility/Simulink-PS Converter  PhysicalDomain=network_engine_domain  SubClassName=ps_input  LeftPortType=input  RightPortType=output  PseudoPeriodic=off  Frequencies=[]  NoiseDistribution=none  NoiseParameters=[]  Unit=1  AffineConversion=off  InputFiltering=on  SimscapeFilterOrder=2  InputFilterTimeConstant=0.001  UdotUserProvided=2
  Simulink-PS Converter5 : nesl_utility/Simulink-PS Converter  PhysicalDomain=network_engine_domain  SubClassName=ps_input  LeftPortType=input  RightPortType=output  PseudoPeriodic=off  Frequencies=[]  NoiseDistribution=none  NoiseParameters=[]  Unit=1  AffineConversion=off  InputFiltering=on  SimscapeFilterOrder=2  InputFilterTimeConstant=0.001  UdotUserProvided=2
  To Workspace : ToWorkspace  VariableName=ankle_trans_out  SaveFormat=Structure With Time  SampleTime=-1
  To Workspace1 : ToWorkspace  VariableName=angle_ie_out  SaveFormat=Structure With Time  SampleTime=-1
  To Workspace2 : ToWorkspace  VariableName=angle_dp_out  SaveFormat=Structure With Time  SampleTime=-1
  To Workspace3 : ToWorkspace  VariableName=tt_ie  SaveFormat=Structure With Time  SampleTime=-1
  To Workspace4 : ToWorkspace  VariableName=tt_dp  SaveFormat=Structure With Time  SampleTime=-1
  To Workspace6 : ToWorkspace  VariableName=acc_ie  SaveFormat=Structure With Time  SampleTime=-1
  To Workspace7 : ToWorkspace  VariableName=vel_ie  SaveFormat=Structure With Time  SampleTime=-1
  To Workspace8 : ToWorkspace  VariableName=acc_dp  SaveFormat=Structure With Time  SampleTime=-1
  To Workspace9 : ToWorkspace  VariableName=vel_dp  SaveFormat=Structure With Time  SampleTime=-1
  Transform Sensor1 : sm_lib/Frames and Transforms/Transform Sensor  MeasurementFrame=Base  SenseAngle=off  SenseAxis=off  SenseAngle1=off  SenseAngle2=off  SenseAngle3=off  SenseQ=off  SenseR=off  SenseOmegaX=off  SenseOmegaY=off  SenseOmegaZ=off  SenseOmega1=off  SenseOmega2=off  SenseOmega3=off  SenseQDot=off  SenseRDot=off  SenseAlphaX=off  SenseAlphaY=off  SenseAlphaZ=off  SenseAlpha1=off  SenseAlpha2=off  SenseAlpha3=off  SenseQDDot=off  SenseRDDot=off  SenseX=on  SenseY=on  SenseZ=on  SenseRad=off  SenseAzim=off  SenseDist=off  SenseInc=off  SenseXDot=off  SenseYDot=off  SenseZDot=off  SenseRadDot=off  SenseAzimDot=off  SenseDistDot=off  SenseIncDot=off  SenseXDDot=off  SenseYDDot=off  SenseZDDot=off  SenseRadDDot=off  SenseAzimDDot=off  SenseDistDDot=off  SenseIncDDot=off
  Transform Sensor2 : sm_lib/Frames and Transforms/Transform Sensor  MeasurementFrame=Base  SenseAngle=off  SenseAxis=off  SenseAngle1=off  SenseAngle2=off  SenseAngle3=off  SenseQ=off  SenseR=on  SenseOmegaX=off  SenseOmegaY=off  SenseOmegaZ=off  SenseOmega1=off  SenseOmega2=off  SenseOmega3=off  SenseQDot=off  SenseRDot=off  SenseAlphaX=off  SenseAlphaY=off  SenseAlphaZ=off  SenseAlpha1=off  SenseAlpha2=off  SenseAlpha3=off  SenseQDDot=off  SenseRDDot=off  SenseX=on  SenseY=on  SenseZ=on  SenseRad=off  SenseAzim=off  SenseDist=off  SenseInc=off  SenseXDot=off  SenseYDot=off  SenseZDot=off  SenseRadDot=off  SenseAzimDot=off  SenseDistDot=off  SenseIncDot=off  SenseXDDot=off  SenseYDDot=off  SenseZDDot=off  SenseRadDDot=off  SenseAzimDDot=off  SenseDistDDot=off  SenseIncDDot=off
  Transform Sensor3 : sm_lib/Frames and Transforms/Transform Sensor  MeasurementFrame=Base  SenseAngle=off  SenseAxis=off  SenseAngle1=off  SenseAngle2=off  SenseAngle3=off  SenseQ=off  SenseR=on  SenseOmegaX=off  SenseOmegaY=off  SenseOmegaZ=off  SenseOmega1=off  SenseOmega2=off  SenseOmega3=off  SenseQDot=off  SenseRDot=off  SenseAlphaX=off  SenseAlphaY=off  SenseAlphaZ=off  SenseAlpha1=off  SenseAlpha2=off  SenseAlpha3=off  SenseQDDot=off  SenseRDDot=off  SenseX=on  SenseY=on  SenseZ=on  SenseRad=off  SenseAzim=off  SenseDist=off  SenseInc=off  SenseXDot=off  SenseYDot=off  SenseZDot=off  SenseRadDot=off  SenseAzimDot=off  SenseDistDot=off  SenseIncDot=off  SenseXDDot=off  SenseYDDot=off  SenseZDDot=off  SenseRadDDot=off  SenseAzimDDot=off  SenseDistDDot=off  SenseIncDDot=off
  Transform Sensor4 : sm_lib/Frames and Transforms/Transform Sensor  MeasurementFrame=Base  SenseAngle=off  SenseAxis=off  SenseAngle1=off  SenseAngle2=off  SenseAngle3=off  SenseQ=on  SenseR=off  SenseOmegaX=on  SenseOmegaY=on  SenseOmegaZ=on  SenseOmega1=off  SenseOmega2=off  SenseOmega3=off  SenseQDot=off  SenseRDot=off  SenseAlphaX=on  SenseAlphaY=on  SenseAlphaZ=on  SenseAlpha1=off  SenseAlpha2=off  SenseAlpha3=off  SenseQDDot=off  SenseRDDot=off  SenseX=off  SenseY=off  SenseZ=off  SenseRad=off  SenseAzim=off  SenseDist=off  SenseInc=off  SenseXDot=off  SenseYDot=off  SenseZDot=off  SenseRadDot=off  SenseAzimDot=off  SenseDistDot=off  SenseIncDot=off  SenseXDDot=off  SenseYDDot=off  SenseZDDot=off  SenseRadDDot=off  SenseAzimDDot=off  SenseDistDDot=off  SenseIncDDot=off
  World : sm_lib/Frames and Transforms/World Frame
  ankle_dp : sm_lib/Joints/Revolute Joint  SenseConstraintForce=off  SenseConstraintForceX=off  SenseConstraintForceY=off  SenseConstraintForceZ=off  SenseConstraintTorque=on  SenseConstraintTorqueX=off  SenseConstraintTorqueY=off  SenseConstraintTorqueZ=off  SenseTotalForce=on  SenseTotalForceX=off  SenseTotalForceY=off  SenseTotalForceZ=off  SenseTotalTorque=on  SenseTotalTorqueX=off  SenseTotalTorqueY=off  SenseTotalTorqueZ=off  CompositeWrenchDir=FollowerOnBase  CompositeWrenchFrame=BaseFrame  EquilibriumPosition=0  EquilibriumPositionUnits=rad  SpringStiffness=stiff_dp  SpringStiffnessUnits=m*N/rad  DampingCoefficient=damp_dp  DampingCoefficientUnits=m*s*N/rad  TorqueActuationMode=InputTorque  MotionActuationMode=ComputedMotion  SensePosition=on  SenseVelocity=on  SenseAcceleration=on  SenseTorqueForce=on  PositionTargetSpecify=off  PositionTargetPriority=Low  PositionTargetValue=-90  PositionTargetValueUnits=deg  VelocityTargetSpecify=off  VelocityTargetPriority=High  VelocityTargetValue=0  VelocityTargetValueUnits=deg/s
  ankle_ie : sm_lib/Joints/Revolute Joint  SenseConstraintForce=off  SenseConstraintForceX=off  SenseConstraintForceY=off  SenseConstraintForceZ=off  SenseConstraintTorque=on  SenseConstraintTorqueX=off  SenseConstraintTorqueY=off  SenseConstraintTorqueZ=off  SenseTotalForce=on  SenseTotalForceX=off  SenseTotalForceY=off  SenseTotalForceZ=off  SenseTotalTorque=on  SenseTotalTorqueX=off  SenseTotalTorqueY=off  SenseTotalTorqueZ=off  CompositeWrenchDir=FollowerOnBase  CompositeWrenchFrame=BaseFrame  EquilibriumPosition=0  EquilibriumPositionUnits=rad  SpringStiffness=stiff_ie  SpringStiffnessUnits=N*m/rad  DampingCoefficient=damp_ie  DampingCoefficientUnits=m*s*N/rad  TorqueActuationMode=InputTorque  MotionActuationMode=ComputedMotion  SensePosition=on  SenseVelocity=on  SenseAcceleration=on  SenseTorqueForce=on  PositionTargetSpecify=off  PositionTargetPriority=Low  PositionTargetValue=0  PositionTargetValueUnits=deg  VelocityTargetSpecify=off  VelocityTargetPriority=High  VelocityTargetValue=0  VelocityTargetValueUnits=deg/s
  ankle_uj1_6_RIGID1 : Subsystem
  ankle_uj1_7_RIGID2 : Subsystem
  ankle_uj2_2_RIGID1 : Subsystem
  foot centre : sm_lib/Frames and Transforms/Reference Frame
  foot tip : sm_lib/Frames and Transforms/Reference Frame
  foot_base_1_RIGID2 : Subsystem
  ft_dp : Scope
  ft_ie : Scope
  motor_knee_1_RIGID : Subsystem
  simple_shin_1_RIGID : Subsystem
  t_dp : Scope
  t_ie : Scope
  tc_dp : Scope
  tc_ie : Scope
  tt_dp : Scope
  tt_ie : Scope
  hip motor : PMIOPort  Port=1  Side=Right
  foot_surface : PMIOPort  Port=2  Side=Right
  f6 : PMIOPort  Port=3  Side=Right
  world : PMIOPort  Port=4  Side=Left
  ie_pos : Outport
  dp_pos : Outport  Port=2
  ie_force : Outport  Port=3
  ie_tor : Outport  Port=4
  dp_tor : Outport  Port=5
  dp_force : Outport  Port=6
  R_ankle : Outport  Port=7
  T_ankle : Outport  Port=8
  dp_vel : Outport  Port=9
  dp_acc : Outport  Port=10
  ie_vel : Outport  Port=11
  ie_acc : Outport  Port=12
  quat_f : Outport  Port=13
  w_f : Outport  Port=14
  b_f : Outport  Port=15
  wires:
  PS-Simulink Converter1/1 -> dp_pos/1, To Workspace2/1
  PS-Simulink Converter4/1 -> ie_vel/1, To Workspace7/1
  PS-Simulink Converter5/1 -> dp_vel/1, To Workspace9/1
  PS-Simulink Converter8/1 -> dp_acc/1, To Workspace8/1
  PS-Simulink Converter9/1 -> Mux/1
  PS-Simulink Converter10/1 -> Mux/2
  PS-Simulink Converter11/1 -> Mux/3
  Mux/1 -> Display1/1
  ankle_ml_tor/1 -> Simulink-PS Converter5/1
  PS-Simulink Converter2/1 -> Display/1
  PS-Simulink Converter3/1 -> ie_pos/1, To Workspace1/1
  ankle_dp_tor/1 -> Simulink-PS Converter/1
  PS-Simulink Converter/1 -> Mux1/1
  PS-Simulink Converter7/1 -> Mux1/2
  PS-Simulink Converter12/1 -> Mux1/3
  Mux1/1 -> To Workspace/1
  PS-Simulink Converter13/1 -> ie_tor/1, tt_ie/1, To Workspace3/1
  PS-Simulink Converter14/1 -> dp_tor/1, tt_dp/1, To Workspace4/1
  PS-Simulink Converter18/1 -> tc_dp/1
  PS-Simulink Converter17/1 -> t_dp/1
  PS-Simulink Converter15/1 -> tc_ie/1
  PS-Simulink Converter16/1 -> t_ie/1
  ankle_ie_tor/1 -> Simulink-PS Converter1/1
  PS-Simulink Converter19/1 -> ft_dp/1, dp_force/1
  PS-Simulink Converter21/1 -> ft_ie/1, ie_force/1
  PS-Simulink Converter26/1 -> Mux2/2
  PS-Simulink Converter25/1 -> Mux2/3
  PS-Simulink Converter24/1 -> Mux2/1
  Mux2/1 -> Display3/1, T_ankle/1
  PS-Simulink Converter27/1 -> Display2/1, R_ankle/1
  PS-Simulink Converter6/1 -> ie_acc/1, To Workspace6/1
  PS-Simulink Converter20/1 -> quat_f/1
  PS-Simulink Converter22/1 -> Mux3/1
  PS-Simulink Converter23/1 -> Mux3/2
  PS-Simulink Converter28/1 -> Mux3/3
  Mux3/1 -> w_f/1
  PS-Simulink Converter29/1 -> Mux4/1
  PS-Simulink Converter30/1 -> Mux4/2
  PS-Simulink Converter31/1 -> Mux4/3
  Mux4/1 -> b_f/1
  connections:
  ankle_uj2_2_RIGID1/LConn1 -- Rigid Transform5/RConn1
  Rigid Transform1/RConn1 -- ankle_dp/LConn1
  simple_shin_1_RIGID/LConn1 -- Rigid Transform/RConn1
  Rigid Transform/LConn1 -- motor_knee_1_RIGID/RConn2
  ankle_uj2_2_RIGID1/RConn1 -- Rigid Transform1/LConn1
  Hip motor/RConn1 -- Transform Sensor2/LConn1 -- motor_knee_1_RIGID/RConn1 -- Frame6/RConn1 -- f6/RConn1
  Hip motor/LConn1 -- hip motor/RConn1
  PS-Simulink Converter4/LConn1 -- ankle_ie/RConn3
  PS-Simulink Converter5/LConn1 -- ankle_dp/RConn3
  PS-Simulink Converter6/LConn1 -- ankle_ie/RConn4
  PS-Simulink Converter8/LConn1 -- ankle_dp/RConn4
  foot_base_1_RIGID2/LConn1 -- ankle_uj1_7_RIGID2/RConn1
  ankle_uj1_7_RIGID2/LConn1 -- ankle_dp/RConn1
  foot_base_1_RIGID2/LConn2 -- Rigid Transform7/LConn1 -- Rigid Transform6/LConn1
  PS-Simulink Converter3/LConn1 -- ankle_ie/RConn2
  PS-Simulink Converter1/LConn1 -- ankle_dp/RConn2
  Transform Sensor2/RConn2 -- PS-Simulink Converter2/LConn1
  Transform Sensor2/RConn3 -- PS-Simulink Converter9/LConn1
  Transform Sensor2/RConn4 -- PS-Simulink Converter10/LConn1
  Transform Sensor2/RConn5 -- PS-Simulink Converter11/LConn1
  Framee/RConn1 -- Transform Sensor3/RConn1 -- Transform Sensor1/RConn1 -- Rigid Transform2/RConn1
  simple_shin_1_RIGID/RConn1 -- ankle_uj1_6_RIGID1/LConn1
  Transform Sensor1/RConn2 -- PS-Simulink Converter/LConn1
  Transform Sensor1/RConn3 -- PS-Simulink Converter7/LConn1
  Transform Sensor1/RConn4 -- PS-Simulink Converter12/LConn1
  ankle_ie/RConn6 -- PS-Simulink Converter15/LConn1
  ankle_ie/RConn5 -- PS-Simulink Converter16/LConn1
  ankle_dp/RConn5 -- PS-Simulink Converter17/LConn1
  ankle_dp/RConn6 -- PS-Simulink Converter18/LConn1
  Rigid Transform2/LConn1 -- ankle_uj1_6_RIGID1/RConn1 -- Rigid Transform4/LConn1
  Rigid Transform4/RConn1 -- Transform Sensor2/RConn1 -- ankle_ie/LConn1
  Rigid Transform5/LConn1 -- ankle_ie/RConn1
  ankle_dp/LConn2 -- Simulink-PS Converter/RConn1
  world/RConn1 -- Transform Sensor4/LConn1 -- Transform Sensor3/LConn1 -- Rigid Transform3/LConn1 -- foot_base_1_RIGID2/LConn3 -- simple_shin_1_RIGID/LConn2
  Hip motor/LConn2 -- Simulink-PS Converter5/RConn1
  ankle_ie/LConn2 -- Simulink-PS Converter1/RConn1
  PS-Simulink Converter14/LConn1 -- ankle_dp/RConn8
  PS-Simulink Converter19/LConn1 -- ankle_dp/RConn7
  Rigid Transform6/RConn1 -- foot tip/RConn1
  Transform Sensor1/LConn1 -- Rigid Transform3/RConn1
  ankle_ie/RConn8 -- PS-Simulink Converter13/LConn1
  ankle_ie/RConn7 -- PS-Simulink Converter21/LConn1
  Rigid Transform7/RConn1 -- Transform Sensor4/RConn1 -- Rigid Transform8/LConn1 -- foot centre/RConn1
  PS-Simulink Converter24/LConn1 -- Transform Sensor3/RConn3
  PS-Simulink Converter26/LConn1 -- Transform Sensor3/RConn4
  PS-Simulink Converter25/LConn1 -- Transform Sensor3/RConn5
  PS-Simulink Converter27/LConn1 -- Transform Sensor3/RConn2
  foot_surface/RConn1 -- Rigid Transform8/RConn1
  Transform Sensor4/RConn5 -- PS-Simulink Converter28/LConn1
  Transform Sensor4/RConn8 -- PS-Simulink Converter31/LConn1
  Transform Sensor4/RConn3 -- PS-Simulink Converter22/LConn1
  Transform Sensor4/RConn6 -- PS-Simulink Converter29/LConn1
  Transform Sensor4/RConn2 -- PS-Simulink Converter20/LConn1
  Transform Sensor4/RConn4 -- PS-Simulink Converter23/LConn1
  Transform Sensor4/RConn7 -- PS-Simulink Converter30/LConn1

== system Impcont_foot/Gait Emulator/Walkway & force plate ==
  fp_dp : Inport
  fp_ie : Inport  Port=2
  FP Contact : Subsystem
  Force Plate : Subsystem
  Ground Contact : Subsystem
  Simulink-PS Converter3 : nesl_utility/Simulink-PS Converter  PhysicalDomain=network_engine_domain  SubClassName=ps_input  LeftPortType=input  RightPortType=output  PseudoPeriodic=off  Frequencies=[]  NoiseDistribution=none  NoiseParameters=[]  Unit=1  AffineConversion=off  InputFiltering=on  SimscapeFilterOrder=2  InputFilterTimeConstant=0.001  UdotUserProvided=1
  Simulink-PS Converter7 : nesl_utility/Simulink-PS Converter  PhysicalDomain=network_engine_domain  SubClassName=ps_input  LeftPortType=input  RightPortType=output  PseudoPeriodic=off  Frequencies=[]  NoiseDistribution=none  NoiseParameters=[]  Unit=1  AffineConversion=off  InputFiltering=on  SimscapeFilterOrder=2  InputFilterTimeConstant=0.0001  UdotUserProvided=1
  Transform2 : sm_lib/Frames and Transforms/Rigid Transform  TranslationMethod=StandardAxis  TranslationLengthUnit=m  TranslationStandardAxis=+Y  TranslationStandardOffset=0.1517  TranslationCartesianOffset=[0 0 0]  TranslationROffset=0  TranslationROffsetUnits=m  TranslationZOffset=0  TranslationZOffsetUnits=m  TranslationThetaOffset=0  TranslationThetaOffsetUnits=deg  RotationMethod=StandardAxis  RotationAngleUnits=deg  RotationStandardAxis=+X  RotationAngle=-90  RotationArbitraryAxis=[0 0 1]  FollAlignAxisA=+X  BaseAlignAxisA=+Y  FollAlignAxisB=+Y  BaseAlignAxisB=+Z  RotationSequenceAxes=FollowerAxes  RotationSequence=XYX  RotationSequenceAngles=[0 0 0]  RotationSequenceAnglesUnits=deg  RotationMatrix=[1 0 0; 0 1 0; 0 0 1]
  walkway_1_RIGID : Subsystem
  world : PMIOPort  Port=1  Side=Left
  foot surface : PMIOPort  Port=2  Side=Right
  fp_force : Outport
  fp_torque : Outport  Port=2
  grn_tor : Outport  Port=3
  fp_tor : Outport  Port=4
  grn_F_f : Outport  Port=5
  grn_T_f : Outport  Port=6
  fp_F_f : Outport  Port=7
  fp_T_f : Outport  Port=8
  wires:
  fp_dp/1 -> Simulink-PS Converter3/1
  fp_ie/1 -> Simulink-PS Converter7/1
  Force Plate/1(fp_force) -> fp_force/1
  Force Plate/2(fp_torque) -> fp_torque/1
  Ground Contact/1(grn_tor) -> grn_tor/1
  FP Contact/1(fp_tor) -> fp_tor/1
  Ground Contact/2(grn_F_f) -> grn_F_f/1
  Ground Contact/3(grn_T_f) -> grn_T_f/1
  FP Contact/3(fp_T_f) -> fp_T_f/1
  FP Contact/2(fp_F_f) -> fp_F_f/1
  connections:
  Force Plate/RConn1 -- FP Contact/RConn1
  FP Contact/LConn1 -- Ground Contact/LConn1 -- foot surface/RConn1
  Ground Contact/RConn1 -- Transform2/RConn1
  Simulink-PS Converter3/RConn1 -- Force Plate/LConn2
  Force Plate/LConn3 -- Simulink-PS Converter7/RConn1
  Transform2/LConn1 -- walkway_1_RIGID/LConn1 -- Force Plate/LConn1 -- world/RConn1

== system Impcont_foot/Gait Emulator/Y Control ==
  inv_kin_y : Inport
  ground force : Inport  Port=2
  Y pos fdbk : Inport  Port=3
  Constant : Constant  Value=0
  PID Controller2 : simulink/Continuous/PID Controller  Controller=PID  TimeDomain=Continuous-time  SampleTime=-1  IntegratorMethod=Forward Euler  FilterMethod=Forward Euler  Form=Parallel  UseFilter=on  ControllerParametersSource=internal  P=81311.420853362  I=160476.881141818  D=5207.81218139461  N=8271.05073782612  InitialConditionSource=internal  InitialConditionForIntegrator=0  InitialConditionForFilter=0  ExternalReset=none  LimitOutput=on  UpperSaturationLimit=2*75*9.81  LowerSaturationLimit=-2*75*9.81  LinearizeAsGain=on  AntiWindupMode=clamping  Kb=1  TrackingMode=off  Kt=1  PParamMin=[]  PParamMax=[]  IParamMin=[]  IParamMax=[]  DParamMin=[]  DParamMax=[]  NParamMin=[]  NParamMax=[]  KbParamMin=[]  KbParamMax=[]  KtParamMin=[]  KtParamMax=[]  POutMin=[]  POutMax=[]  IOutMin=[]  IOutMax=[]  DOutMin=[]  DOutMax=[]  NOutMin=[]  NOutMax=[]  KbOutMin=[]  KbOutMax=[]  KtOutMin=[]  KtOutMax=[]  IntegratorOutMin=[]  IntegratorOutMax=[]  FilterOutMin=[]  FilterOutMax=[]  SumOutMin=[]  SumOutMax=[]  SumI1OutMin=[]  SumI1OutMax=[]  SumI2OutMin=[]  SumI2OutMax=[]  SumI3OutMin=[]  SumI3OutMax=[]  SumDOutMin=[]  SumDOutMax=[]  SaturationOutMin=[]  SaturationOutMax=[]  IntegratorContinuousStateAttributes=''  IntegratorStateMustResolveToSignalObject=off  IntegratorRTWStateStorageClass=Auto  FilterContinuousStateAttributes=''  FilterStateMustResolveToSignalObject=off  FilterRTWStateStorageClass=Auto  DifferentiatorICPrevScaledInput=0  DifferentiatorOutMin=[]  DifferentiatorOutMax=[]
  Sum3 : Sum  Inputs=|+-
  Switch1 : Switch  Criteria=u2 > Threshold
  Y for : Outport
  wires:
  Y pos fdbk/1 -> Sum3/2
  Constant/1 -> Switch1/1
  Sum3/1 -> PID Controller2/1
  PID Controller2/1 -> Switch1/3
  inv_kin_y/1 -> Sum3/1
  Switch1/1 -> Y for/1
  ground force/1 -> Switch1/2
